simulink model "IPMSMAxleDriveEVDQ"  (R2025b)
settings: Solver=VariableStepAuto  StartTime=0.0  StopTime=2  RelTol=1e-3  EnableMultiTasking=on
PreLoadFcn:
  | IPMSMAxleDriveEVDQData;
values from neighbouring files (symbols this model uses):
  AL = 0.9    [IPMSMAxleDriveEVDQData.m]
  Cd = 0.4    [IPMSMAxleDriveEVDQData.m]
  cr1 = 0.1    [IPMSMAxleDriveEVDQData.m]
  cr2 = 0.2    [IPMSMAxleDriveEVDQData.m]
  g = 9.8    [IPMSMAxleDriveEVDQData.m]
  i_t = 9    [IPMSMAxleDriveEVDQData.m]
  Ki_id = 710.3004    [IPMSMAxleDriveEVDQData.m]
  Ki_iq = 1.0615e+03    (= 1061.5)    [IPMSMAxleDriveEVDQData.m]
  Kp_id = 0.8779    [IPMSMAxleDriveEVDQData.m]
  Kp_iq = 1.0744    [IPMSMAxleDriveEVDQData.m]
  Ld = 0.00024368    [IPMSMAxleDriveEVDQData.m]
  Lq = 0.00029758    [IPMSMAxleDriveEVDQData.m]
  Mv = 1100    [IPMSMAxleDriveEVDQData.m]
  p = 8    [IPMSMAxleDriveEVDQData.m]
  psim = 0.04366    [IPMSMAxleDriveEVDQData.m]
  rho_a = 1.2    [IPMSMAxleDriveEVDQData.m]
  Rw = 0.3    [IPMSMAxleDriveEVDQData.m]
  Tmax = 205    [IPMSMAxleDriveEVDQData.m]
libraries: fl_lib x59, nesl_utility x13, eeDiscretePi x2, batteryecm_lib x1, eeDqVoltageLimiter x1, eePmsmCurrentReferenceGen x1, eePmsmTorqueEstimator x1, ee_lib x1, SignalEditorBlockLib x1
CloseFcn:
  | try,close(h1_IPMSMAxleDriveEVDQ),end
  | clear h1_IPMSMAxleDriveEVDQ
  | 
  | clear simlog_IPMSMAxleDriveEVDQ
  | clear logsout_IPMSMAxleDriveEVDQ
  | 
  | 
  | clear Pmax Tmax p psim Ld Lq L0 Rs Jm
  | clear Cdc Vnom V1 AH0
  | clear Ts fsw Tsi Kp_id Ki_id Kp_iq Ki_iq
  | clear numd_id dend_id numd_iq dend_iq
  | clear ID_MAP IQ_MAP RPM_VECT TQ_VECT VDC_VECT
  | clear Mv g rho_a AL Cd cr1 cr2 i_t Rw
Description:
  | Control Torque of IPMSM Inside Axle-Drive EV in DQ Frame
settings Model: Creator=The MathWorks, Inc.  LastModifiedBy=adity
settings SolverCC: AlgebraicLoopSolver=TrustRegion  MaxZcPerStep=1.0
settings DataIOCC: MaxDataPoints=510000  SaveOutput=off  SignalLogging=off  SaveTime=off  ReturnWorkspaceOutputs=off
settings OptimizationCC: ReuseModelBlockBuffer=off  LifeSpan=inf
settings DebuggingCC: UnderspecifiedInitializationDetection=Classic  MergeDetectMultiDrivingBlocksExec=none  UnconnectedInputMsg=warning  UnconnectedOutputMsg=warning  UnconnectedLineMsg=warning  SFUnexpectedBacktrackingDiag=warning  SFNoUnconditionalDefaultTransitionDiag=warning  SFExecutionAtInitializationDiag=none  ArithmeticOperatorsInVariantConditions=warning
settings ModelReferenceCC: EnableRefExpFcnMdlSchedulingChecks=on
settings SFSimCC: SimUseLocalCustomCode=off  CustomCodeUndefinedFunction=UseInterfaceOnly
settings RTWCC: RTWUseLocalCustomCode=off  GPUComputeCapability=3.5  DLArmComputeVersion=19.05
settings CodeAppCC: StateflowObjectComments=on
settings GRTTargetCC: TargetLangStandard=C89/C90 (ANSI)
settings ConfigComp: CovMetricSettings=dw  CovSaveCumulativeToWorkspaceVar=on  CovSaveSingleToWorkspaceVar=on  CovExternalEMLEnable=off
settings SimscapeCC: SimscapeNormalizeSystem=off  SimscapeLogType=all  SimscapeLogSimulationStatistics=on  SimscapeLogName=simlog_IPMSMAxleDriveEVDQ  SimscapeLogDataHistory=510000.0

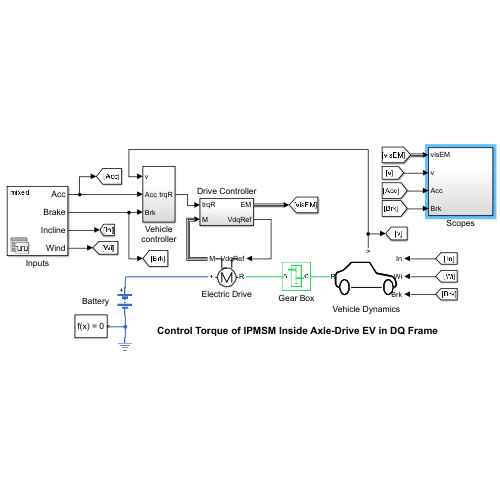
[thumbnail: Simulink's stored preview of the top-level diagram]
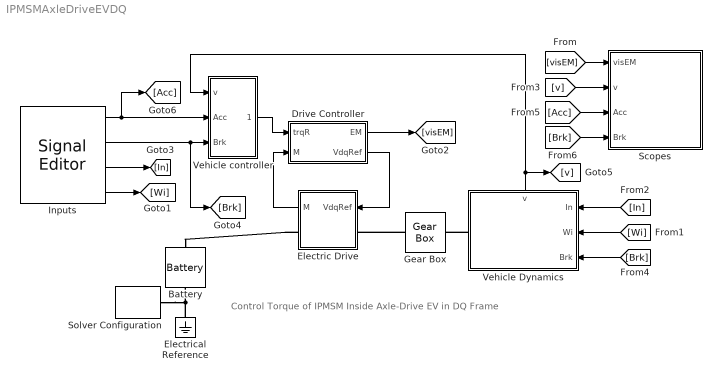
== system IPMSMAxleDriveEVDQ ==
  note: Control Torque of IPMSM Inside Axle-Drive EV in DQ Frame
  Battery : batteryecm_lib/Battery  Vnom=Vnom V  prm_dir=1  R1_dis=2 Ohm  R1_ch=2 Ohm  R1=0.001 Ohm  prm_AH=1  AH=300 hr*A  V1=V1 V  AH1=100 hr*A  prm_R2=1  R2=2000 Ohm  Tmeas=298.15 K  charge_measurement_port=simscape.enum.battery.enable.no  prm_dyn=1  Rp1=0.005 Ohm  tau1=30 s  Rp2=0.005 Ohm  tau2=30 s  Rp3=0.005 Ohm  tau3=30 s  Rp4=0.005 Ohm  tau4=30 s  Rp5=0.005 Ohm  tau5=30 s  prm_fade=1  N_fade=100  AH_fade=45 hr*A  R1_fade=2.02 Ohm  R1_ch_fade=2.02 Ohm  V1_fade=10.35 V  prm_age=1  prm_age_OCV=1  OCV_age=0.9  SOC_age=60  Tmeas_age=298.15 K  delta_time_age_vec=[0] d  temperature_age_vec=[273] K  OCV_scaling_age=2.2134e6  OCV_offset_age=1.632e6  temp_exp_age=0.515833569 V  t_exp_age=0.75  Vnom_T2=12 V  R1_T2=2.2 Ohm  R1_T2_dis=2.2 Ohm  R1_T2_ch=2.2 Ohm  V1_T2=11.4 V  R2_T2=2200 Ohm  Rp1_T2=0.005 Ohm  tau1_T2=30 s  Rp2_T2=0.005 Ohm  tau2_T2=30 s  Rp3_T2=0.005 Ohm  tau3_T2=30 s  Rp4_T2=0.005 Ohm  tau4_T2=30 s  Rp5_T2=0.005 Ohm  tau5_T2=30 s  Tmeas2=273.15 K  thermal_port=simscape.enum.thermaleffects.omit  thermal_mass=30000 J/K  i_specify=off  i_priority=None  i=0 A  i_nominal_specify=off  i_nominal_value=1  i_nominal_unit=A  v_specify=off  v_priority=None  v=0 V  v_nominal_specify=off  v_nominal_value=1  v_nominal_unit=V  charge_specify=on  charge_priority=High  charge=AH0 hr*A  charge_nominal_specify=off  charge_nominal_value=1  charge_nominal_unit=A*hr  num_cycles_specify=off  num_cycles_priority=High  num_cycles=0  num_cycles_nominal_specify=off  num_cycles_nominal_value=1  num_cycles_nominal_unit=1  temperature_specify=off  temperature_priority=High  temperature=298.15 K  temperature_nominal_specify=off  temperature_nominal_value=1  temperature_nominal_unit=K
  Drive Controller : Subsystem
  Electric Drive : Subsystem  Tag=PublishSubsystem
      mask Display:
      | % Circle
      | plot(sin(0:0.1:2.2*pi)*0.9,cos(0:0.1:2.2*pi)*0.9);
      | 
      | % In/out
      | plot([-1.1 -0.9],[0 0]);
      | plot([1.1 0.9],[0 0]);
      | 
      | % 'M'
      | plot([0.5 0.5],[-0.5 0.5]);
      | plot([-0.5 -0.5],[-0.5 0.5]);
      | plot([0.5 0],[0.5 -0.5]);
      | plot([-0.5 0],[0.5 -0.5]);
      | 
      | % Inputs and Outputs
      | plot([0.5 0.5],[0.9 1.8]);
      | plot([0.5 1.1],[1.8 1.8]);
      | 
      | plot([-0.5 -0.5],[0.9 1.8]);
      | plot([-0.5 -1.1],[1.8 1.8]);
      | 
      | 
      | % Plot points to set plot range
      | color('white');plot(1.9,2.8);plot(-1.9,0)
      | color('black');
  Electrical Reference : fl_lib/Electrical/Electrical Elements/Electrical Reference
  Gear Box : fl_lib/Mechanical/Mechanisms/Gear Box  ratio=i_t  t_in_specify=off  t_in_priority=None  t_in=0 N*m  t_in_nominal_specify=off  t_in_nominal_value=1  t_in_nominal_unit=N*m  t_out_specify=off  t_out_priority=None  t_out=0 N*m  t_out_nominal_specify=off  t_out_nominal_value=1  t_out_nominal_unit=N*m
  Inputs : SignalEditorBlockLib/Signal Editor  FileName=IPMSMAxleDriveEVInputs.mat  ActiveScenario=mixed  ActiveSignal=Wind  IsBus=off  OutputBusObjectStr=Bus: BusObject  SampleTime=0  OutputAfterFinalValue=Extrapolation  Unit=inherit  PreserveSignalName=on  ApplySigPropsToAllScenarios=on  ApplySigPropsToAllSignals=off  SignalPropertySource=Dialog parameters
  Scopes : Subsystem
  Solver Configuration : nesl_utility/Solver Configuration  PhysicalDomain=network_engine_domain  SubClassName=solver  LeftPortType=input  RightPortType=generic  Tones=[]  Harmonics=[]  SimulateNoise=off  Profile=off  UseLocalSampling=off  EnableSwitchedLinearOptims=on  FrequencyDomain=off  UseCCode=off  RelTol=0.001  AbsTol=0.001  MinStep=1e-09  ToWorkspace=off  RevertToSquareIcSolve=off  NumHomotopyIterations=100  PhasorMode=off  PhasorModeNumHarmonics=1  ConsistencySolver=NEWTON_XTOL_AFTER_FTOL  IndexReductionMethod=DerivativeReplacement  DoDC=off  ResidualTolerance=1e-09  ConsistencyTolSource=GLOBAL  ConsistencyAbsTol=0.001  ConsistencyRelTol=0.001  ConsistencyTolFactor=0.001  UseLocalSolver=off  LocalSolverChoice=NE_BACKWARD_EULER_ADVANCER  ResolveIndetEquations=on  FunctionEvalNumThread=1  LocalSolverSampleTime=0.001  DoFixedCost=off  MaxNonlinIter=3  MaxModeIter=2  ComputeImpulses=off  ImpulseIterations=2  LinearAlgebra=auto  LinearAlgebraNumThread=0  EquationFormulation=NE_TIME_EF  DelaysMemoryBudget=1024  AutomaticFiltering=on  FilteringTimeConstant=0.001  PartitionStorageMethod=AS_NEEDED  PartitionMemoryBudget=1024  PartitionMethod=ROBUST  MultibodyUseLocalSolver=off  MultibodyLocalSolverChoice=ODE1  MultibodyLocalSolverSampleTime=0.001
  Vehicle controller : Subsystem
  Vehicle Dynamics : Subsystem
      settings: PortSchema="{\"entries\":[{\"content\":{\"sides\":[{\"content\":{\"connectorIds\":[\"In1\",\"In2\",\"In3\"]},\"type\":\"ConnectorPlacement.EquallySpacedRectSide\",\"uuid\":\"e4001960-f2e0-4b02-b30e-a2c6bf4e04d0\"},{\"content\":{\"connectorIds\":[\"RConn1\"],\"side\":\"RIGHT\"},\"type\":\"ConnectorPlacement.EquallySpacedRectSide\",\"uuid\":\"dc10d66e-73c4-4edd-a023-0857b4dc6f5e\"},{\"content\":{\"connectorIds\":[\"Out1\"],\"side\":\"TOP\"},\"type\":\"ConnectorPlacement.EquallySpacedRectSide\",\"uuid\":\"bb7ebb83-0e11-4294-ba38-25417a0ec075\"}]},\"type\":\"ConnectorPlacement.EquallySpacedConnector\",\"uuid\":\"5d34a695-2a89-4153-bca5-b4c38ec60820\"}],\"packageUris\":[\"http://schema.mathworks.com/mf0/Connector/R2020b\"],\"version\":\"1.0\"}"
      mask Display:
      | color('white')
      | plot(-120,-60); plot(120,50);
      | color('black')
      | plot(sin(0:0.1:6*pi)*15-70,cos(0:0.1:6*pi)*15-30);
      | plot(sin(0:0.1:6*pi)*15+70,cos(0:0.1:6*pi)*15-30);
      | plot([-88 -95 -99 -99 -95 -75 -65 -50 -46 10 30 34 80 85 90 93 95 93 90 88],[-30 -28 -23 -5 0 5 10 20 21 21 0 -2 -7 -9 -13 -17 -25 -28 -30 -30])
      | plot([-88 -95 -99 -99 -95 -75 -65 -50 -46 10 30 34 80 85 90 93 95 93 90 88],[-30 -28 -23 -5 0 5 10 20 21 21 0 -2 -7 -9 -13 -17 -25 -28 -30 -30]-1)
      | plot([-88 -95 -99 -99 -95 -75 -65 -50 -46 10 30 34 80 85 90 93 95 93 90 88]+1,[-30 -28 -23 -5 0 5 10 20 21 21 0 -2 -7 -9 -13 -17 -25 -28 -30 -30])
      | plot([-50 50],[-30 -30])
  wires:
  Vehicle controller/1(trqR) -> Drive Controller/1(trqR)
  Electric Drive/1(M) -> Drive Controller/2(M)
  [Wi] -> Vehicle Dynamics/2(Wi)
  Drive Controller/2(VdqRef) -> Electric Drive/1(VdqRef)
  Inputs/3 -> [In]
  [Brk] -> Vehicle Dynamics/3(Brk)
  [In] -> Vehicle Dynamics/1(In)
  Inputs/1 -> [Acc], Vehicle controller/2(Acc)
  Inputs/2 -> [Brk], Vehicle controller/3(Brk)
  Inputs/4 -> [Wi]
  Drive Controller/1(EM) -> [visEM]
  [visEM] -> Scopes/1(visEM)
  Vehicle Dynamics/1(v) -> Vehicle controller/1(v), [v]
  [v] -> Scopes/2(v)
  [Acc] -> Scopes/3(Acc)
  [Brk] -> Scopes/4(Brk)
  connections:
  Battery/RConn1 -- Solver Configuration/RConn1 -- Electrical Reference/LConn1
  Electric Drive/RConn1 -- Battery/LConn1
  Gear Box/LConn1 -- Electric Drive/LConn1
  Vehicle Dynamics/RConn1 -- Gear Box/RConn1

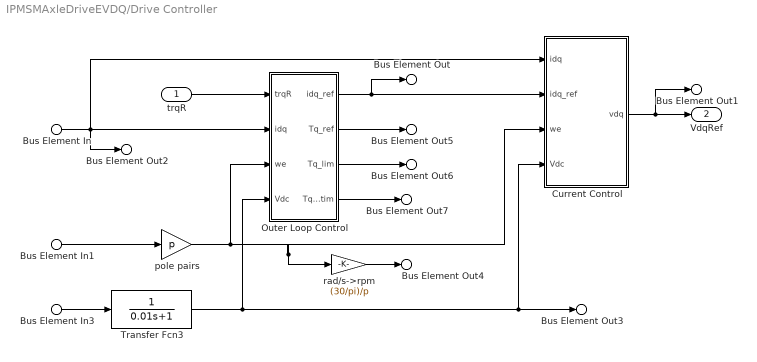
== system IPMSMAxleDriveEVDQ/Drive Controller ==
  trqR : Inport
  Bus Element In : Inport  Port=2  PortName=M  Element=idq
  Bus Element In1 : Inport  Port=2  PortName=M  Element=w
  Bus Element In3 : Inport  Port=2  PortName=M  Element=vdc
  Current Control : Subsystem
  Outer Loop Control : Subsystem
  Transfer Fcn3 : TransferFcn  Denominator=[0.01 1]
  pole pairs : Gain  Gain=p
  rad/s->rpm : Gain  Gain=(30/pi)/p
  Bus Element Out : Outport  PortName=EM  Element=idqRef
  Bus Element Out1 : Outport  PortName=EM  Element=vdq
  Bus Element Out2 : Outport  PortName=EM  Element=idq
  Bus Element Out3 : Outport  PortName=EM  Element=vdc
  Bus Element Out4 : Outport  PortName=EM  Element=rpm
  Bus Element Out5 : Outport  PortName=EM  Element=trqR
  Bus Element Out6 : Outport  PortName=EM  Element=trqLim
  Bus Element Out7 : Outport  PortName=EM  Element=trqEst
  VdqRef : Outport  Port=2  VectorParamsAs1DForOutWhenUnconnected=off
  wires:
  Outer Loop Control/2(Tq_ref) -> Bus Element Out5/1
  Bus Element In/1 -> Bus Element Out2/1, Outer Loop Control/2(idq), Current Control/1(idq)
  Outer Loop Control/3(Tq_lim) -> Bus Element Out6/1
  Transfer Fcn3/1 -> Bus Element Out3/1, Current Control/4(Vdc), Outer Loop Control/4(Vdc)
  Outer Loop Control/1(idq_ref) -> Current Control/2(idq_ref), Bus Element Out/1
  pole pairs/1 -> rad/s->rpm/1, Current Control/3(we), Outer Loop Control/3(we)
  rad/s->rpm/1 -> Bus Element Out4/1
  trqR/1 -> Outer Loop Control/1(trqR)
  Current Control/1(vdq) -> VdqRef/1, Bus Element Out1/1
  Bus Element In3/1 -> Transfer Fcn3/1
  Bus Element In1/1 -> pole pairs/1
  Outer Loop Control/4(Tq_estim) -> Bus Element Out7/1

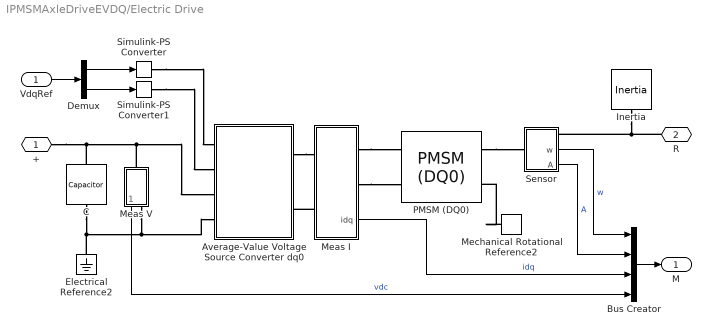
== system IPMSMAxleDriveEVDQ/Electric Drive ==
  VdqRef : Inport
  Average-Value Voltage Source Converter dq0 : Subsystem
  Bus Creator : BusCreator  Inputs=4
  C : fl_lib/Electrical/Electrical Elements/Capacitor  c=Cdc F  r=0 Ohm  g=0 1/Ohm  i_specify=off  i_priority=None  i=0 A  i_nominal_specify=off  i_nominal_value=1  i_nominal_unit=A  v_specify=off  v_priority=None  v=0 V  v_nominal_specify=off  v_nominal_value=1  v_nominal_unit=V  vc_specify=on  vc_priority=None  vc=Vnom V  vc_nominal_specify=off  vc_nominal_value=1  vc_nominal_unit=V
  Demux : Demux  Outputs=2
  Electrical Reference2 : fl_lib/Electrical/Electrical Elements/Electrical Reference
  Inertia : fl_lib/Mechanical/Rotational Elements/Inertia  inertia=Jm kg*m^2  num_ports=foundation.enum.numPorts2.one  w_specify=off  w_priority=High  w=0 rad/s  w_nominal_specify=off  w_nominal_value=1  w_nominal_unit=rad/s  t_specify=off  t_priority=None  t=0 N*m  t_nominal_specify=off  t_nominal_value=1  t_nominal_unit=N*m
  Meas I : Subsystem
      settings: PortSchema="{\"entries\":[{\"content\":{\"sides\":[{\"content\":{\"connectorIds\":[\"LConn1\",\"LConn2\"]},\"type\":\"ConnectorPlacement.EquallySpacedRectSide\",\"uuid\":\"3a4028b2-8937-42a6-80f4-68b1695ce77d\"},{\"content\":{\"connectorIds\":[\"RConn1\",\"RConn2\",\"Out1\"],\"side\":\"RIGHT\"},\"type\":\"ConnectorPlacement.EquallySpacedRectSide\",\"uuid\":\"b0265b90-0b10-444b-91c2-8367167e2f75\"},{\"content\":{\"side\":\"TOP\"},\"type\":\"ConnectorPlacement.EquallySpacedRectSide\",\"uuid\":\"a56d3a18-e083-4f19-8a6c-1d5eb0dcfc62\"}]},\"type\":\"ConnectorPlacement.EquallySpacedConnector\",\"uuid\":\"f333dc84-7c1b-47f0-a9ed-bc0e1c61b934\"}],\"packageUris\":[\"http://schema.mathworks.com/mf0/Connector/R2020b\"],\"version\":\"1.0\"}"
      mask Display: %disp('iABC');
  Meas V : Subsystem
  Mechanical Rotational Reference2 : fl_lib/Mechanical/Rotational Elements/Mechanical Rotational Reference
  PMSM (DQ0) : ee_lib/Electromechanical/Permanent Magnet/PMSM (DQ0)  machine_param=ee.enum.pmsm.parameterization.constant  nPolePairs=p  pmflux_param=ee.enum.pmflux.fluxlinkage  pm_flux_linkage=psim Wb  torque_constant=0.18 N*m/A  back_emf_constant=0.18 V*s/rad  stator_param=ee.enum.statorparam.LdLqL0  Ld=Ld H  Lq=Lq H  idVec=[-200, 0, 200] A  iqVec=[-200, 0, 200] A  LdMatrix=0.0002 * ones(3, 3) H  LqMatrix=0.0002 * ones(3, 3) H  PmMatrix=0.1 * ones(3, 3) Wb  ktMatrix=0.18 * ones(3, 3) N*m/A  keMatrix=0.18 * ones(3, 3) V*s/rad  L0=0.00016 H  Ls=0.0002 H  Lm=-0.00002 H  Ms=0.00002 H  Rs=Rs Ohm  zero_sequence=ee.enum.park.zerosequence.exclude  loss_param=ee.enum.ironloss.none  losses_oc=[0, 0, 0] W  losses_sc=[0, 0, 0] W  f_losses=60 Hz  Isc_losses=95 A  J=0 kg*m^2  lam=0 N*m*s/rad  i_d_specify=off  i_d_priority=None  i_d=0 A  i_d_nominal_specify=off  i_d_nominal_value=1  i_d_nominal_unit=A  i_q_specify=off  i_q_priority=None  i_q=0 A  i_q_nominal_specify=off  i_q_nominal_value=1  i_q_nominal_unit=A  torque_specify=off  torque_priority=None  torque=0 N*m  torque_nominal_specify=off  torque_nominal_value=1  torque_nominal_unit=N*m  angular_velocity_specify=on  angular_velocity_priority=None  angular_velocity=0 rpm  angular_velocity_nominal_specify=off  angular_velocity_nominal_value=1  angular_velocity_nominal_unit=rpm  angular_position_specify=off  angular_position_priority=High  angular_position=0 deg  angular_position_nominal_specify=off  angular_position_nominal_value=1  angular_position_nominal_unit=deg  alpha=3.93e-3 1/K  alpha_flux=-0.001 1/K  Tmeas=298.15 K  stator_thermal_mass=100 J/K  rotor_thermal_mass=200 J/K  Rm_percent_rotor=90  Rd_percent_rotor=30  temperatureS_specify=off  temperatureS_priority=High  temperatureS=25 degC  temperatureS_nominal_specify=off  temperatureS_nominal_value=1  temperatureS_nominal_unit=degC  temperatureR_specify=off  temperatureR_priority=High  temperatureR=25 degC  temperatureR_nominal_specify=off  temperatureR_nominal_value=1  temperatureR_nominal_unit=degC
      settings: InternalSimscapePortConfiguration="{\"Bottom\":[],\"Left\":[{\"id\":\"d\",\"label\":\"D\",\"type\":\"foundation.electrical.electrical\"},{\"id\":\"q\",\"label\":\"Q\",\"type\":\"foundation.electrical.electrical\"}],\"Right\":[{\"id\":\"R\",\"label\":\"R\",\"type\":\"foundation.mechanical.rotational.rotational\"},{\"id\":\"C\",\"label\":\"C\",\"type\":\"foundation.mechanical.rotational.rotational\"}],\"Top\":[]}"
  Sensor : Subsystem
      settings: PortSchema="{\"entries\":[{\"content\":{\"sides\":[{\"content\":{\"connectorIds\":[\"LConn1\"]},\"type\":\"ConnectorPlacement.EquallySpacedRectSide\",\"uuid\":\"9716bd1c-b62c-4027-b550-f14c70f36db1\"},{\"content\":{\"connectorIds\":[\"RConn1\",\"Out1\",\"Out2\"],\"side\":\"RIGHT\"},\"type\":\"ConnectorPlacement.EquallySpacedRectSide\",\"uuid\":\"da6cfd9e-9128-4eb3-99c5-1cd2bc57b3d6\"},{\"content\":{\"side\":\"TOP\"},\"type\":\"ConnectorPlacement.EquallySpacedRectSide\",\"uuid\":\"dd7de32f-f9ca-4ba4-8a93-24a44c04d88b\"}]},\"type\":\"ConnectorPlacement.EquallySpacedConnector\",\"uuid\":\"7e726746-2fa5-4a48-8428-e3741c603e47\"}],\"packageUris\":[\"http://schema.mathworks.com/mf0/Connector/R2020b\"],\"version\":\"1.0\"}"
  Simulink-PS Converter : nesl_utility/Simulink-PS Converter  PhysicalDomain=network_engine_domain  SubClassName=ps_input  LeftPortType=input  RightPortType=output  PseudoPeriodic=off  Frequencies=[]  NoiseDistribution=none  NoiseParameters=[]  Unit=V  AffineConversion=off  FilteringAndDerivatives=provide  SimscapeFilterOrder=1  InputFilterTimeConstant=0.001  UdotUserProvided=0
  Simulink-PS Converter1 : nesl_utility/Simulink-PS Converter  PhysicalDomain=network_engine_domain  SubClassName=ps_input  LeftPortType=input  RightPortType=output  PseudoPeriodic=off  Frequencies=[]  NoiseDistribution=none  NoiseParameters=[]  Unit=V  AffineConversion=off  FilteringAndDerivatives=provide  SimscapeFilterOrder=1  InputFilterTimeConstant=0.001  UdotUserProvided=0
  + : PMIOPort  Side=Right
  R : PMIOPort  Port=2  Side=Left
  M : Outport  VectorParamsAs1DForOutWhenUnconnected=off
  wires:
  Bus Creator/1 -> M/1
  Meas I/1(idq) -> Bus Creator/3  "idq"
  Sensor/1(w) -> Bus Creator/1  "w"
  Sensor/2(A) -> Bus Creator/2  "A"
  Meas V/1(Vdc) -> Bus Creator/4  "vdc"
  VdqRef/1 -> Demux/1
  Demux/1 -> Simulink-PS Converter/1
  Demux/2 -> Simulink-PS Converter1/1
  connections:
  Meas I/RConn1 -- PMSM (DQ0)/LConn1
  R/RConn1 -- Sensor/RConn1 -- Inertia/LConn1
  +/RConn1 -- C/LConn1 -- Average-Value Voltage Source Converter dq0/LConn3 -- Meas V/LConn1
  Electrical Reference2/LConn1 -- C/RConn1 -- Meas V/RConn1 -- Average-Value Voltage Source Converter dq0/LConn4
  Mechanical Rotational Reference2/LConn1 -- PMSM (DQ0)/RConn2
  PMSM (DQ0)/RConn1 -- Sensor/LConn1
  Average-Value Voltage Source Converter dq0/RConn1 -- Meas I/LConn1
  Meas I/LConn2 -- Average-Value Voltage Source Converter dq0/RConn2
  Meas I/RConn2 -- PMSM (DQ0)/LConn2
  Simulink-PS Converter/RConn1 -- Average-Value Voltage Source Converter dq0/LConn1
  Simulink-PS Converter1/RConn1 -- Average-Value Voltage Source Converter dq0/LConn2

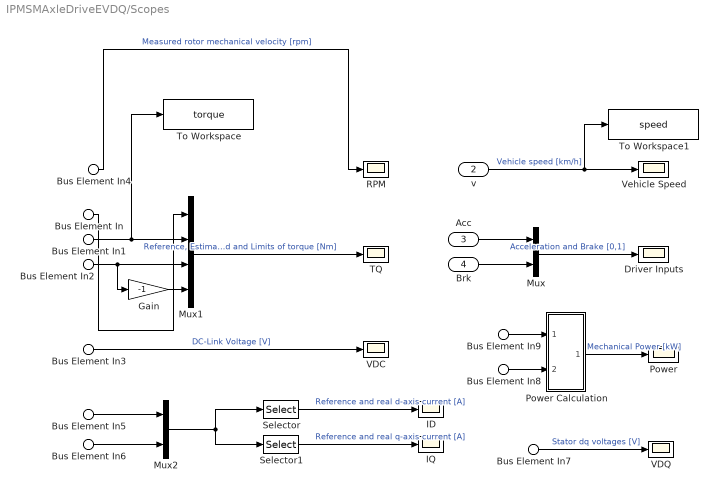
== system IPMSMAxleDriveEVDQ/Scopes ==
  Bus Element In : Inport  PortName=visEM  Element=trqR
  Bus Element In1 : Inport  PortName=visEM  Element=trqEst
  Bus Element In8 : Inport  PortName=visEM  Element=trqEst
  Bus Element In2 : Inport  PortName=visEM  Element=trqLim
  Bus Element In3 : Inport  PortName=visEM  Element=vdc
  Bus Element In4 : Inport  PortName=visEM  Element=rpm
  Bus Element In9 : Inport  PortName=visEM  Element=rpm
  Bus Element In5 : Inport  PortName=visEM  Element=idqRef
  Bus Element In6 : Inport  PortName=visEM  Element=idq
  Bus Element In7 : Inport  PortName=visEM  Element=vdq
  v : Inport  Port=2
  Acc : Inport  Port=3
  Brk : Inport  Port=4
  Driver Inputs : Scope
      settings: ActiveDisplayYMinimum=-0.12499999999999997  ActiveDisplayYMaximum=1.125  DataLoggingVariableName=ScopeData2
  Gain : Gain  Gain=-1
  ID : Scope
      settings: ActiveDisplayYMinimum=-139.0162  ActiveDisplayYMaximum=16.19169  DataLoggingVariableName=ScopeData4  DataLoggingSaveFormat=Array
  IQ : Scope
      settings: ActiveDisplayYMinimum=-43.36566  ActiveDisplayYMaximum=382.05756  DataLoggingVariableName=ScopeData5  DataLoggingSaveFormat=Array
  Mux : Mux  Inputs=2
  Mux1 : Mux
  Mux2 : Mux  Inputs=2
  Power : Scope
      settings: ActiveDisplayYMinimum=-44.20842  ActiveDisplayYMaximum=43.99515  DataLoggingVariableName=ScopeData6
  Power Calculation : Subsystem
  RPM : Scope
      settings: ActiveDisplayYMinimum=-887.33768266130551  ActiveDisplayYMaximum=3417.5586307610274  DataLoggingVariableName=ScopeData8
  Selector : Selector  InputPortWidth=4  IndexOptions=Index vector (dialog)  Indices=[1 3]  OutputSizes=1
  Selector1 : Selector  InputPortWidth=4  IndexOptions=Index vector (dialog)  Indices=[2 4]  OutputSizes=1
  TQ : Scope
      settings: ActiveDisplayYMinimum=-272.00900256295347  ActiveDisplayYMaximum=266.39448631176469  DataLoggingVariableName=ScopeData10
  To Workspace : ToWorkspace  VariableName=torque  SampleTime=-1
      settings: Save2DSignal=2-D array (concatenate along first dimension)
  To Workspace1 : ToWorkspace  VariableName=speed  SampleTime=-1
      settings: Save2DSignal=2-D array (concatenate along first dimension)
  VDC : Scope
      settings: ActiveDisplayYMinimum=-40.636621495100485  ActiveDisplayYMaximum=365.72959345590442  DataLoggingVariableName=ScopeData11
  VDQ : Scope
      settings: ActiveDisplayYMinimum=-203.83105  ActiveDisplayYMaximum=198.95882  DataLoggingVariableName=ScopeData12
  Vehicle Speed : Scope
      settings: ActiveDisplayYMinimum=-3.5625978626211872  ActiveDisplayYMaximum=32.063380763590693
  wires:
  Power Calculation/1(Power) -> Power/1  "Mechanical Power [kW]"
  Gain/1 -> Mux1/4
  Bus Element In6/1 -> Mux2/2
  Bus Element In9/1 -> Power Calculation/1(rpm)
  Bus Element In5/1 -> Mux2/1
  v/1 -> Vehicle Speed/1, To Workspace1/1  "Vehicle speed [km/h]"
  Mux1/1 -> TQ/1  "Reference, Estimated and Limits of torque [Nm]"
  Bus Element In7/1 -> VDQ/1  "Stator dq voltages [V]"
  Bus Element In/1 -> Mux1/1
  Bus Element In2/1 -> Mux1/3, Gain/1
  Selector/1 -> ID/1  "Reference and real d-axis current [A]"
  Mux2/1 -> Selector1/1, Selector/1
  Mux/1 -> Driver Inputs/1  "Acceleration and Brake [0,1]"
  Selector1/1 -> IQ/1  "Reference and real q-axis current [A]"
  Brk/1 -> Mux/2
  Acc/1 -> Mux/1
  Bus Element In4/1 -> RPM/1  "Measured rotor mechanical velocity [rpm]"
  Bus Element In3/1 -> VDC/1  "DC-Link Voltage [V]"
  Bus Element In8/1 -> Power Calculation/2(Tq)
  Bus Element In1/1 -> Mux1/2, To Workspace/1

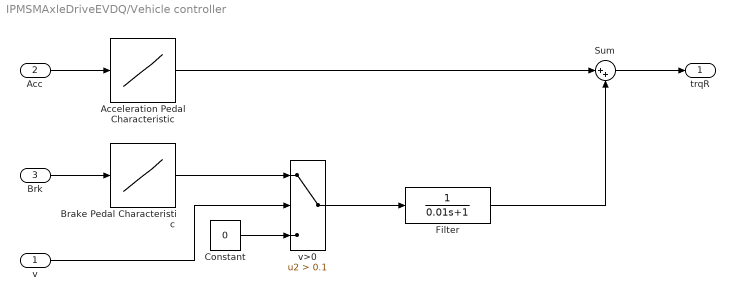
== system IPMSMAxleDriveEVDQ/Vehicle controller ==
  v : Inport
  Acc : Inport  Port=2
  Brk : Inport  Port=3
  Acceleration Pedal Characteristic : Lookup_n-D  NumberOfTableDimensions=1  BreakpointsForDimension1=0:0.1:1  Table=[0 0.04 0.07 0.1 0.16 0.2 0.3 0.4 0.6 0.8 1]*Tmax  InternalRulePriority=Speed  RndMeth=Simplest
  Brake Pedal Characteristic : Lookup_n-D  NumberOfTableDimensions=1  BreakpointsForDimension1=[0 0.03 0.04 0.3 0.4 0.5 0.6 0.7 0.8 0.9 1]  Table=[0 0 0.04 0.05 0.06 0.2 0.25 0.4 0.6 0.8 1]*(-Tmax)  InternalRulePriority=Speed  RndMeth=Simplest
  Constant : Constant  Value=0
  Filter : TransferFcn  Denominator=[0.01 1]
  Sum : Sum  Inputs=|++
  v>0 : Switch  Criteria=u2 > Threshold  Threshold=0.1  SaturateOnIntegerOverflow=off  InputSameDT=off
  trqR : Outport  VectorParamsAs1DForOutWhenUnconnected=off
  wires:
  Sum/1 -> trqR/1
  Filter/1 -> Sum/2
  v/1 -> v>0/2
  v>0/1 -> Filter/1
  Constant/1 -> v>0/3
  Brake Pedal Characteristic/1 -> v>0/1
  Acceleration Pedal Characteristic/1 -> Sum/1
  Brk/1 -> Brake Pedal Characteristic/1
  Acc/1 -> Acceleration Pedal Characteristic/1

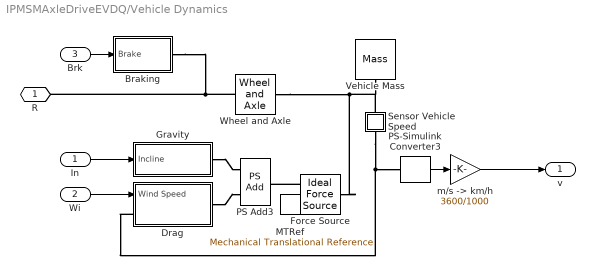
== system IPMSMAxleDriveEVDQ/Vehicle Dynamics ==
  In : Inport
  Wi : Inport  Port=2
  Brk : Inport  Port=3
  Braking : Subsystem
  Drag : Subsystem
  Force Source : fl_lib/Mechanical/Mechanical Sources/Ideal Force Source
  Gravity : Subsystem
  MTRef : fl_lib/Mechanical/Translational Elements/Mechanical Translational Reference
  PS Add3 : fl_lib/Physical Signals/Functions/PS Add
  PS-Simulink Converter3 : nesl_utility/PS-Simulink Converter  PhysicalDomain=network_engine_domain  SubClassName=ps_output  LeftPortType=input  RightPortType=output  PseudoPeriodic=off  Frequencies=[]  VectorFormat=1-D array  Unit=m/s  AffineConversion=off
  Sensor Vehicle Speed : Subsystem
      mask Display: disp('v')
  Vehicle Mass : fl_lib/Mechanical/Translational Elements/Mass  mass=Mv kg  num_ports=foundation.enum.numPorts2.one  v_specify=off  v_priority=High  v=0 m/s  v_nominal_specify=off  v_nominal_value=1  v_nominal_unit=m/s  f_specify=off  f_priority=None  f=0 N  f_nominal_specify=off  f_nominal_value=1  f_nominal_unit=N
  Wheel and Axle : fl_lib/Mechanical/Mechanisms/Wheel and Axle  R=Rw m  or=1  t_specify=off  t_priority=None  t=0 N*m  t_nominal_specify=off  t_nominal_value=1  t_nominal_unit=N*m  f_specify=off  f_priority=None  f=0 N  f_nominal_specify=off  f_nominal_value=1  f_nominal_unit=N
  "m/s -> km/h" : Gain  Gain=3600/1000
  R : PMIOPort  Side=Right
  v : Outport
  wires:
  PS-Simulink Converter3/1 -> "m/s -> km/h"/1
  "m/s -> km/h"/1 -> v/1
  Brk/1 -> Braking/1(Brake)
  Wi/1 -> Drag/1(Wind Speed)
  In/1 -> Gravity/1(Incline)
  connections:
  Wheel and Axle/LConn1 -- Braking/RConn1 -- R/RConn1
  MTRef/LConn1 -- Force Source/RConn2
  Drag/RConn1 -- PS Add3/LConn2
  Gravity/RConn1 -- PS Add3/LConn1
  Force Source/RConn1 -- PS Add3/RConn1
  Drag/LConn1 -- Sensor Vehicle Speed/RConn1 -- PS-Simulink Converter3/LConn1
  Wheel and Axle/RConn1 -- Vehicle Mass/LConn1 -- Sensor Vehicle Speed/LConn1 -- Force Source/LConn1

== system IPMSMAxleDriveEVDQ/Drive Controller/Current Control ==
  idq : Inport
  idq_ref : Inport  Port=2
  we : Inport  Port=3
  Vdc : Inport  Port=4
  Constant : Constant  Value=0
  Current controller : Subsystem
  Gain : Gain  Gain=1/sqrt(3)
  vdq : Outport  VectorParamsAs1DForOutWhenUnconnected=off
  wires:
  idq/1 -> Current controller/2(idq)
  Vdc/1 -> Gain/1
  we/1 -> Current controller/3(wElectrical)
  idq_ref/1 -> Current controller/1(idqRef)
  Constant/1 -> Current controller/5(Reset)
  Gain/1 -> Current controller/4(VphMax)
  Current controller/1(vdqRef) -> vdq/1

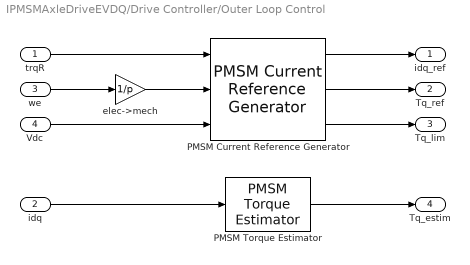
== system IPMSMAxleDriveEVDQ/Drive Controller/Outer Loop Control ==
  trqR : Inport
  idq : Inport  Port=2
  we : Inport  Port=3
  Vdc : Inport  Port=4
  PMSM Current Reference Generator : eePmsmCurrentReferenceGen/PMSM Current Reference Generator  Vnom=Vnom  Pmax=Pmax  Tmax=Tmax  Ts=0  RefType=Lookup-table based  rpmVec=RPM_VECT  TqVec=TQ_VECT  VdcVec=VDC_VECT  PWMMode=SVM: space vector modulation  ModFactor=1  idMatrix=ID_MAP  iqMatrix=IQ_MAP  p=8  psim=0.04  Ld=0.00024  Lq=0.00029  Rs=0.01  RefExpEnable=0
  PMSM Torque Estimator : eePmsmTorqueEstimator/PMSM Torque Estimator  ParamType=Constant parameters  p=p  idVect=[-200, 200]  iqVect=[-200, 200]  LdMatrix=0.0002 * ones(2, 2)  LqMatrix=0.0002 * ones(2, 2)  psimMatrix=0.04 * ones(2, 2)  Ld=Ld  Lq=Lq  psim=psim  Ts=0
  elec->mech : Gain  Gain=1/p
  idq_ref : Outport  VectorParamsAs1DForOutWhenUnconnected=off
  Tq_ref : Outport  Port=2  VectorParamsAs1DForOutWhenUnconnected=off
  Tq_lim : Outport  Port=3  VectorParamsAs1DForOutWhenUnconnected=off
  Tq_estim : Outport  Port=4  VectorParamsAs1DForOutWhenUnconnected=off
  wires:
  idq/1 -> PMSM Torque Estimator/1
  PMSM Current Reference Generator/2 -> Tq_ref/1
  PMSM Current Reference Generator/1 -> idq_ref/1
  Vdc/1 -> PMSM Current Reference Generator/3
  elec->mech/1 -> PMSM Current Reference Generator/2
  trqR/1 -> PMSM Current Reference Generator/1
  PMSM Current Reference Generator/3 -> Tq_lim/1
  we/1 -> elec->mech/1
  PMSM Torque Estimator/1 -> Tq_estim/1

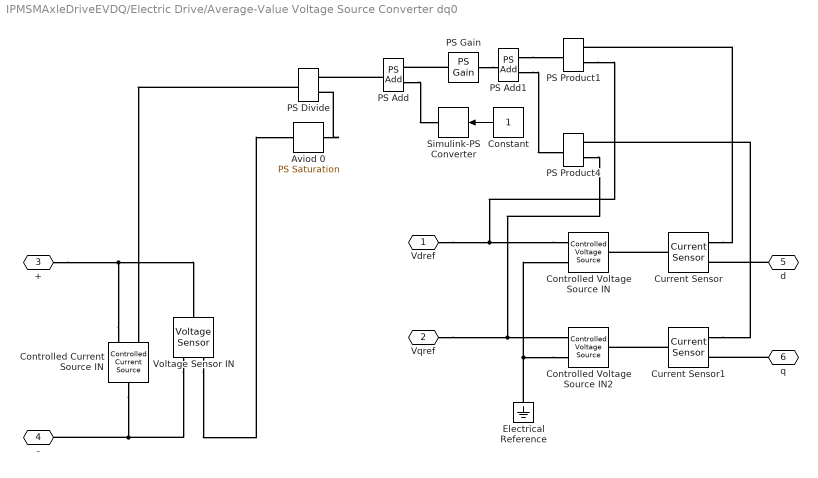
== system IPMSMAxleDriveEVDQ/Electric Drive/Average-Value Voltage Source Converter dq0 ==
  Aviod 0 : fl_lib/Physical Signals/Nonlinear Operators/PS Saturation  upper_limit=inf V  lower_limit=1e-6 V  ZeroCross=true
  Constant : Constant  SampleTime=0
  Controlled Current Source IN : fl_lib/Electrical/Electrical Sources/Controlled Current Source
  Controlled Voltage Source IN : fl_lib/Electrical/Electrical Sources/Controlled Voltage Source
  Controlled Voltage Source IN2 : fl_lib/Electrical/Electrical Sources/Controlled Voltage Source
  Current Sensor : fl_lib/Electrical/Electrical Sensors/Current Sensor
  Current Sensor1 : fl_lib/Electrical/Electrical Sensors/Current Sensor
  Electrical Reference : fl_lib/Electrical/Electrical Elements/Electrical Reference
  PS Add : fl_lib/Physical Signals/Functions/PS Add
  PS Add1 : fl_lib/Physical Signals/Functions/PS Add
  PS Divide : fl_lib/Physical Signals/Functions/PS Divide
  PS Gain : fl_lib/Physical Signals/Functions/PS Gain  gain=3/2
  PS Product1 : fl_lib/Physical Signals/Functions/PS Product
  PS Product4 : fl_lib/Physical Signals/Functions/PS Product
  Simulink-PS Converter : nesl_utility/Simulink-PS Converter  PhysicalDomain=network_engine_domain  SubClassName=ps_input  LeftPortType=input  RightPortType=output  PseudoPeriodic=off  Frequencies=[]  NoiseDistribution=none  NoiseParameters=[]  Unit=W  AffineConversion=off  FilteringAndDerivatives=provide  SimscapeFilterOrder=1  InputFilterTimeConstant=0.001  UdotUserProvided=0
  Voltage Sensor IN : fl_lib/Electrical/Electrical Sensors/Voltage Sensor
  Vdref : PMIOPort  Side=Left
  Vqref : PMIOPort  Port=2  Side=Left
  + : PMIOPort  Port=3  Side=Left
  - : PMIOPort  Port=4  Side=Left
  d : PMIOPort  Port=5  Side=Right
  q : PMIOPort  Port=6  Side=Right
  wires:
  Constant/1 -> Simulink-PS Converter/1
  connections:
  Controlled Current Source IN/RConn2 -- Voltage Sensor IN/LConn1 -- +/RConn1
  -/RConn1 -- Voltage Sensor IN/RConn2 -- Controlled Current Source IN/LConn1
  Controlled Voltage Source IN2/RConn2 -- Electrical Reference/LConn1 -- Controlled Voltage Source IN/RConn2
  Current Sensor1/LConn1 -- Controlled Voltage Source IN2/LConn1
  Current Sensor/LConn1 -- Controlled Voltage Source IN/LConn1
  Voltage Sensor IN/RConn1 -- Aviod 0/LConn1
  Controlled Voltage Source IN/RConn1 -- Vdref/RConn1 -- PS Product1/LConn2
  Vqref/RConn1 -- Controlled Voltage Source IN2/RConn1 -- PS Product4/LConn2
  PS Add1/LConn1 -- PS Product1/RConn1
  PS Add1/LConn2 -- PS Product4/RConn1
  Aviod 0/RConn1 -- PS Divide/LConn2
  PS Divide/RConn1 -- Controlled Current Source IN/RConn1
  PS Add/RConn1 -- PS Divide/LConn1
  PS Add/LConn2 -- Simulink-PS Converter/RConn1
  d/RConn1 -- Current Sensor/RConn2
  q/RConn1 -- Current Sensor1/RConn2
  Current Sensor/RConn1 -- PS Product1/LConn1
  Current Sensor1/RConn1 -- PS Product4/LConn1
  PS Gain/LConn1 -- PS Add1/RConn1
  PS Gain/RConn1 -- PS Add/LConn1

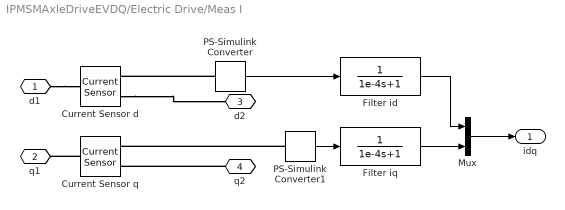
== system IPMSMAxleDriveEVDQ/Electric Drive/Meas I ==
  Current Sensor d : fl_lib/Electrical/Electrical Sensors/Current Sensor
  Current Sensor q : fl_lib/Electrical/Electrical Sensors/Current Sensor
  Filter id : TransferFcn  Denominator=[1e-4 1]
  Filter iq : TransferFcn  Denominator=[1e-4 1]
  Mux : Mux  Inputs=2
  PS-Simulink Converter : nesl_utility/PS-Simulink Converter  PhysicalDomain=network_engine_domain  SubClassName=ps_output  LeftPortType=input  RightPortType=output  PseudoPeriodic=off  Frequencies=[]  VectorFormat=1-D array  Unit=A  AffineConversion=off
  PS-Simulink Converter1 : nesl_utility/PS-Simulink Converter  PhysicalDomain=network_engine_domain  SubClassName=ps_output  LeftPortType=input  RightPortType=output  PseudoPeriodic=off  Frequencies=[]  VectorFormat=1-D array  Unit=A  AffineConversion=off
  d1 : PMIOPort  Side=Left
  q1 : PMIOPort  Port=2  Side=Left
  d2 : PMIOPort  Port=3  Side=Right
  q2 : PMIOPort  Port=4  Side=Right
  idq : Outport  VectorParamsAs1DForOutWhenUnconnected=off
  wires:
  PS-Simulink Converter1/1 -> Filter iq/1
  PS-Simulink Converter/1 -> Filter id/1
  Mux/1 -> idq/1
  Filter id/1 -> Mux/1
  Filter iq/1 -> Mux/2
  connections:
  d1/RConn1 -- Current Sensor d/LConn1
  Current Sensor q/LConn1 -- q1/RConn1
  Current Sensor d/RConn2 -- d2/RConn1
  q2/RConn1 -- Current Sensor q/RConn2
  PS-Simulink Converter/LConn1 -- Current Sensor d/RConn1
  PS-Simulink Converter1/LConn1 -- Current Sensor q/RConn1

== system IPMSMAxleDriveEVDQ/Electric Drive/Meas V ==
  PS-Simulink Converter4 : nesl_utility/PS-Simulink Converter  PhysicalDomain=network_engine_domain  SubClassName=ps_output  LeftPortType=input  RightPortType=output  PseudoPeriodic=off  Frequencies=[]  VectorFormat=1-D array  Unit=V  AffineConversion=off
  Voltage Sensor : fl_lib/Electrical/Electrical Sensors/Voltage Sensor
  - : PMIOPort  Side=Right
  + : PMIOPort  Port=2  Side=Left
  Vdc : Outport  VectorParamsAs1DForOutWhenUnconnected=off
  wires:
  PS-Simulink Converter4/1 -> Vdc/1
  connections:
  PS-Simulink Converter4/LConn1 -- Voltage Sensor/RConn1
  Voltage Sensor/LConn1 -- +/RConn1
  Voltage Sensor/RConn2 -- -/RConn1

== system IPMSMAxleDriveEVDQ/Electric Drive/Sensor ==
  Filter A : TransferFcn  Denominator=[1e-4 1]
  Filter w : TransferFcn  Denominator=[1e-4 1]
  MRRef : fl_lib/Mechanical/Rotational Elements/Mechanical Rotational Reference
  Motion Sensor : fl_lib/Mechanical/Mechanical Sensors/Ideal Rotational Motion Sensor  reference=foundation.enum.MeasurementReference.difference  acceleration_port=false  velocity_port=true  position_port=true  wrap_angle=simscape.enum.onoff.off  offset=0 deg
  PS-Simulink Converter1 : nesl_utility/PS-Simulink Converter  PhysicalDomain=network_engine_domain  SubClassName=ps_output  LeftPortType=input  RightPortType=output  PseudoPeriodic=off  Frequencies=[]  VectorFormat=1-D array  Unit=rad/s  AffineConversion=off
  PS-Simulink Converter2 : nesl_utility/PS-Simulink Converter  PhysicalDomain=network_engine_domain  SubClassName=ps_output  LeftPortType=input  RightPortType=output  PseudoPeriodic=off  Frequencies=[]  VectorFormat=1-D array  Unit=rad  AffineConversion=off
  R : PMIOPort  Side=Left
  C : PMIOPort  Port=2  Side=Right
  w : Outport  VectorParamsAs1DForOutWhenUnconnected=off
  A : Outport  Port=2  VectorParamsAs1DForOutWhenUnconnected=off
  wires:
  PS-Simulink Converter1/1 -> Filter w/1
  PS-Simulink Converter2/1 -> Filter A/1
  Filter A/1 -> A/1
  Filter w/1 -> w/1
  connections:
  Motion Sensor/RConn2 -- PS-Simulink Converter1/LConn1
  Motion Sensor/RConn1 -- MRRef/LConn1
  C/RConn1 -- R/RConn1 -- Motion Sensor/LConn1
  Motion Sensor/RConn3 -- PS-Simulink Converter2/LConn1

== system IPMSMAxleDriveEVDQ/Scopes/Power Calculation ==
  rpm : Inport
  Tq : Inport  Port=2
  Gain3 : Gain  Gain=pi/30
  Gain4 : Gain  Gain=1/1000
  Product2 : Product
  Power : Outport  VectorParamsAs1DForOutWhenUnconnected=off
  wires:
  rpm/1 -> Gain3/1
  Gain4/1 -> Power/1
  Product2/1 -> Gain4/1
  Tq/1 -> Product2/2
  Gain3/1 -> Product2/1

== system IPMSMAxleDriveEVDQ/Vehicle Dynamics/Braking ==
  Brake : Inport
  Lookup Table (1D) : fl_lib/Physical Signals/Lookup Tables/PS Lookup Table (1D)  x=[0 0.03 0.04 0.3 0.4 0.5 0.6 0.7 0.8 0.9 1]  f=[0 0 0.04 0.05 0.06 0.2 0.25 0.4 0.6 0.8 1]*(-Tmax)*i_t N*m  interp_method=simscape.enum.interpolation.linear  extrap_method=simscape.enum.extrapolation.linear
  MRRef : fl_lib/Mechanical/Rotational Elements/Mechanical Rotational Reference
  PS Product : fl_lib/Physical Signals/Functions/PS Product
  PS Terminator : fl_lib/Physical Signals/Sinks/PS Terminator
  Rotational Motion Sensor : fl_lib/Mechanical/Mechanical Sensors/Ideal Rotational Motion Sensor  reference=foundation.enum.MeasurementReference.difference  acceleration_port=false  velocity_port=true  position_port=true  wrap_angle=simscape.enum.onoff.off  offset=0 rad
  Simulink-PS Converter : nesl_utility/Simulink-PS Converter  PhysicalDomain=network_engine_domain  SubClassName=ps_input  LeftPortType=input  RightPortType=output  PseudoPeriodic=off  Frequencies=[]  NoiseDistribution=none  NoiseParameters=[]  Unit=1  AffineConversion=off  FilteringAndDerivatives=filter  SimscapeFilterOrder=1  InputFilterTimeConstant=0.001  UdotUserProvided=1
  Smooth Sign : Subsystem
  Torque Source : fl_lib/Mechanical/Mechanical Sources/Ideal Torque Source
  R : PMIOPort  Side=Right
  wires:
  Brake/1 -> Simulink-PS Converter/1
  connections:
  Torque Source/LConn1 -- Rotational Motion Sensor/LConn1 -- R/RConn1
  PS Product/RConn1 -- Torque Source/RConn1
  MRRef/LConn1 -- Rotational Motion Sensor/RConn1 -- Torque Source/RConn2
  PS Terminator/LConn1 -- Rotational Motion Sensor/RConn3
  Lookup Table (1D)/RConn1 -- PS Product/LConn1
  Simulink-PS Converter/RConn1 -- Lookup Table (1D)/LConn1
  Smooth Sign/LConn1 -- Rotational Motion Sensor/RConn2
  PS Product/LConn2 -- Smooth Sign/RConn1

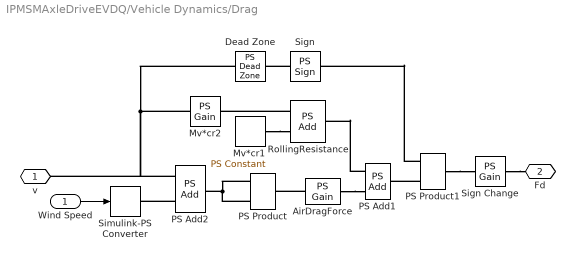
== system IPMSMAxleDriveEVDQ/Vehicle Dynamics/Drag ==
  Wind Speed : Inport
  AirDragForce : fl_lib/Physical Signals/Functions/PS Gain  gain=0.5*rho_a*AL*Cd N/(m/s)^2
  Dead Zone : fl_lib/Physical Signals/Nonlinear Operators/PS Dead Zone  upper_limit=0.1 m/s  lower_limit=-0.001 m/s  ZeroCross=true
      settings: InternalSimscapePortConfiguration="{\"Bottom\":[],\"Left\":[{\"id\":\"I\",\"label\":\"\",\"type\":\"input\"}],\"Right\":[{\"id\":\"O\",\"label\":\"\",\"type\":\"output\"}],\"Top\":[]}"
  Mv*cr1 : fl_lib/Physical Signals/Sources/PS Constant  constant=Mv*cr1 N
  Mv*cr2 : fl_lib/Physical Signals/Functions/PS Gain  gain=Mv*cr2 N/(m/s)
  PS Add1 : fl_lib/Physical Signals/Functions/PS Add
  PS Add2 : fl_lib/Physical Signals/Functions/PS Add
  PS Product : fl_lib/Physical Signals/Functions/PS Product
  PS Product1 : fl_lib/Physical Signals/Functions/PS Product
  RollingResistance : fl_lib/Physical Signals/Functions/PS Add
  Sign : fl_lib/Physical Signals/Nonlinear Operators/PS Sign
      settings: InternalSimscapePortConfiguration="{\"Bottom\":[],\"Left\":[{\"id\":\"I\",\"label\":\"\",\"type\":\"input\"}],\"Right\":[{\"id\":\"O\",\"label\":\"\",\"type\":\"output\"}],\"Top\":[]}"
  Sign Change : fl_lib/Physical Signals/Functions/PS Gain  gain=-1
  Simulink-PS Converter : nesl_utility/Simulink-PS Converter  PhysicalDomain=network_engine_domain  SubClassName=ps_input  LeftPortType=input  RightPortType=output  PseudoPeriodic=off  Frequencies=[]  NoiseDistribution=none  NoiseParameters=[]  Unit=m/s  AffineConversion=off  FilteringAndDerivatives=filter  SimscapeFilterOrder=1  InputFilterTimeConstant=0.001  UdotUserProvided=1
  v : PMIOPort  Side=Left
  Fd : PMIOPort  Port=2  Side=Right
  wires:
  Wind Speed/1 -> Simulink-PS Converter/1
  connections:
  AirDragForce/RConn1 -- PS Add1/LConn2
  PS Product1/LConn2 -- PS Add1/RConn1
  PS Add2/LConn2 -- Simulink-PS Converter/RConn1
  PS Product/LConn1 -- PS Product/LConn2 -- PS Add2/RConn1
  PS Product1/LConn1 -- Sign/RConn1
  Sign Change/RConn1 -- Fd/RConn1
  AirDragForce/LConn1 -- PS Product/RConn1
  PS Add1/LConn1 -- RollingResistance/RConn1
  Mv*cr1/RConn1 -- RollingResistance/LConn2
  Sign/LConn1 -- Dead Zone/RConn1
  RollingResistance/LConn1 -- Mv*cr2/RConn1
  PS Product1/RConn1 -- Sign Change/LConn1
  Dead Zone/LConn1 -- PS Add2/LConn1 -- v/RConn1 -- Mv*cr2/LConn1

== system IPMSMAxleDriveEVDQ/Vehicle Dynamics/Gravity ==
  Incline : Inport
  GravitationalForce : fl_lib/Physical Signals/Functions/PS Gain  gain=-1 N
  Mv*g : fl_lib/Physical Signals/Functions/PS Gain  gain=Mv*g
  Simulink-PS Converter1 : nesl_utility/Simulink-PS Converter  PhysicalDomain=network_engine_domain  SubClassName=ps_input  LeftPortType=input  RightPortType=output  PseudoPeriodic=off  Frequencies=[]  NoiseDistribution=none  NoiseParameters=[]  Unit=rad  AffineConversion=off  FilteringAndDerivatives=filter  SimscapeFilterOrder=1  InputFilterTimeConstant=0.001  UdotUserProvided=1
  deg->rad : Gain  Gain=pi/180
  sin : fl_lib/Physical Signals/Functions/PS Math Function  fcn_choice=1  v=1
  Fg : PMIOPort  Side=Right
  wires:
  Incline/1 -> deg->rad/1
  deg->rad/1 -> Simulink-PS Converter1/1
  connections:
  Simulink-PS Converter1/RConn1 -- sin/LConn1
  Mv*g/LConn1 -- sin/RConn1
  Mv*g/RConn1 -- GravitationalForce/LConn1
  GravitationalForce/RConn1 -- Fg/RConn1

== system IPMSMAxleDriveEVDQ/Vehicle Dynamics/Sensor Vehicle Speed ==
  MTRef15 : fl_lib/Mechanical/Translational Elements/Mechanical Translational Reference
  PS Terminator : fl_lib/Physical Signals/Sinks/PS Terminator
  Translational Motion Sensor : fl_lib/Mechanical/Mechanical Sensors/Ideal Translational Motion Sensor  reference=foundation.enum.MeasurementReference.difference  acceleration_port=false  velocity_port=true  position_port=true  offset=0 m
  Conn1 : PMIOPort  Side=Left
  Conn2 : PMIOPort  Port=2  Side=Right
  connections:
  Translational Motion Sensor/LConn1 -- Conn1/RConn1
  Translational Motion Sensor/RConn1 -- MTRef15/LConn1
  Translational Motion Sensor/RConn2 -- Conn2/RConn1
  Translational Motion Sensor/RConn3 -- PS Terminator/LConn1

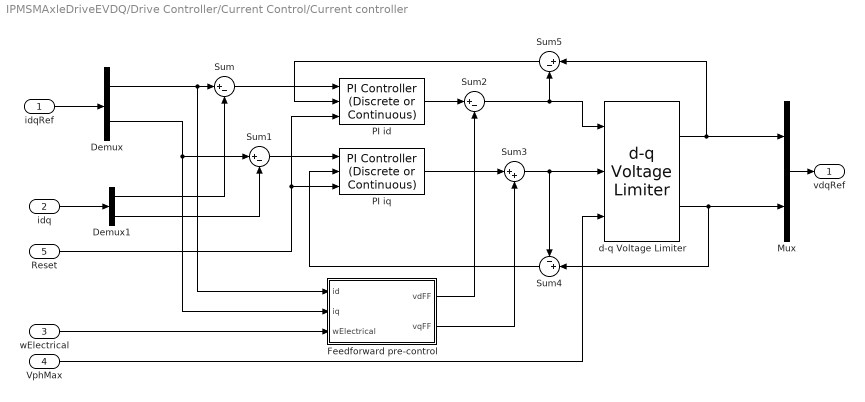
== system IPMSMAxleDriveEVDQ/Drive Controller/Current Control/Current controller ==
  idqRef : Inport
  idq : Inport  Port=2
  wElectrical : Inport  Port=3
  VphMax : Inport  Port=4
  Reset : Inport  Port=5
  Demux : Demux  Outputs=2
  Demux1 : Demux  Outputs=2
  Feedforward pre-control : Subsystem
  Mux : Mux  Inputs=2
  PI id : eeDiscretePi/PI Controller (Discrete or Continuous)  Kp=Kp_id  Ki=Ki_id  Kaw=1  x0=0  Ts=0
  PI iq : eeDiscretePi/PI Controller (Discrete or Continuous)  Kp=Kp_iq  Ki=Ki_iq  Kaw=1  x0=0  Ts=0
  Sum{,1..2,5} (4 alike) : Sum  Inputs=|+-
  Sum3 : Sum  Inputs=|++
  Sum4 : Sum  Inputs=-+|
  d-q Voltage Limiter : eeDqVoltageLimiter/d-q Voltage Limiter  AxisPrio=Q-axis  Ts=0
  vdqRef : Outport  VectorParamsAs1DForOutWhenUnconnected=off
  wires:
  Demux1/1 -> Sum/2
  idq/1 -> Demux1/1
  Demux/2 -> Feedforward pre-control/2(iq), Sum1/1
  Reset/1 -> PI id/3, PI iq/3
  Sum3/1 -> Sum4/1, d-q Voltage Limiter/2
  Sum4/1 -> PI iq/2
  VphMax/1 -> d-q Voltage Limiter/3
  Mux/1 -> vdqRef/1
  Feedforward pre-control/2(vqFF) -> Sum3/2
  wElectrical/1 -> Feedforward pre-control/3(wElectrical)
  idqRef/1 -> Demux/1
  Sum/1 -> PI id/1
  PI id/1 -> Sum2/1
  Sum5/1 -> PI id/2
  PI iq/1 -> Sum3/1
  Feedforward pre-control/1(vdFF) -> Sum2/2
  Sum1/1 -> PI iq/1
  Demux/1 -> Sum/1, Feedforward pre-control/1(id)
  Demux1/2 -> Sum1/2
  Sum2/1 -> Sum5/2, d-q Voltage Limiter/1
  d-q Voltage Limiter/1 -> Mux/1, Sum5/1
  d-q Voltage Limiter/2 -> Mux/2, Sum4/2

== system IPMSMAxleDriveEVDQ/Vehicle Dynamics/Braking/Smooth Sign ==
  1 : fl_lib/Physical Signals/Sources/PS Constant  constant=1
  2 : fl_lib/Physical Signals/Functions/PS Gain  gain=2 s/rad
  exp(2x) : fl_lib/Physical Signals/Functions/PS Math Function  fcn_choice=3  v=1
  exp(2x)+1 : fl_lib/Physical Signals/Functions/PS Add
  exp(2x)-1 : fl_lib/Physical Signals/Functions/PS Subtract
  tanh(x) : fl_lib/Physical Signals/Functions/PS Divide
  x : PMIOPort  Side=Left
  y : PMIOPort  Port=2  Side=Right
  connections:
  y/RConn1 -- tanh(x)/RConn1
  x/RConn1 -- 2/LConn1
  exp(2x)-1/RConn1 -- tanh(x)/LConn1
  exp(2x)+1/RConn1 -- tanh(x)/LConn2
  exp(2x)+1/LConn2 -- exp(2x)-1/LConn1 -- exp(2x)/RConn1
  2/RConn1 -- exp(2x)/LConn1
  exp(2x)-1/LConn2 -- exp(2x)+1/LConn1 -- 1/RConn1

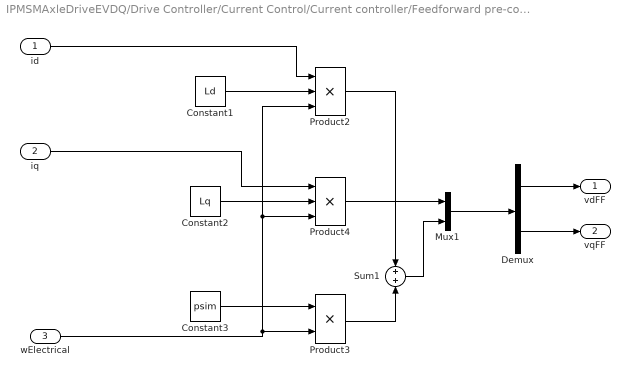
== system IPMSMAxleDriveEVDQ/Drive Controller/Current Control/Current controller/Feedforward pre-control ==
  id : Inport
  iq : Inport  Port=2
  wElectrical : Inport  Port=3
  Constant1 : Constant  Value=Ld
  Constant2 : Constant  Value=Lq
  Constant3 : Constant  Value=psim
  Demux : Demux  Outputs=2
  Mux1 : Mux  Inputs=2
  Product2 : Product  Inputs=3
  Product3 : Product
  Product4 : Product  Inputs=3
  Sum1 : Sum
  vdFF : Outport  VectorParamsAs1DForOutWhenUnconnected=off
  vqFF : Outport  Port=2  VectorParamsAs1DForOutWhenUnconnected=off
  wires:
  Product2/1 -> Sum1/1
  wElectrical/1 -> Product2/3, Product4/3, Product3/2
  Product4/1 -> Mux1/1
  id/1 -> Product2/1
  iq/1 -> Product4/1
  Constant1/1 -> Product2/2
  Sum1/1 -> Mux1/2
  Constant3/1 -> Product3/1
  Demux/2 -> vqFF/1
  Demux/1 -> vdFF/1
  Mux1/1 -> Demux/1
  Constant2/1 -> Product4/2
  Product3/1 -> Sum1/2
